simulink model "Pokus08_Display_2x2"  (Simulink 8.1)
settings: Solver=FixedStepDiscrete  StartTime=0.0  StopTime=10.0  RelTol=1e-3
libraries: simulink_extras x1, Displays_Lib x1, Computer_Library x1
settings Model: Creator=uzivatel  LastModifiedBy=uzivatel
settings DataIOCC: SignalLoggingSaveFormat=Dataset
settings OptimizationCC: ExpressionDepthLimit=128
settings DebuggingCC: FcnCallInpInsideContextMsg=EnableAllAsError
settings GRTTargetCC: CombineOutputUpdateFcns=on  GRTInterface=off

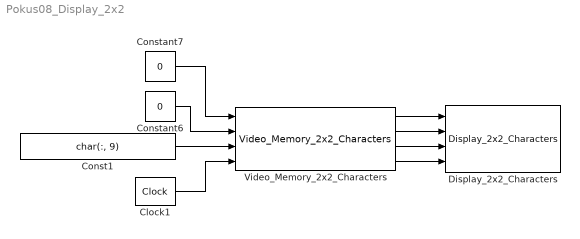
== system Pokus08_Display_2x2 ==
  Clock1 : simulink_extras/Flip Flops/Clock  period=1
  Const1 : Constant  Value=char(:, 9)  OutDataTypeStr=uint8
  Constant6 : Constant  Value=0  OutDataTypeStr=uint8
  Constant7 : Constant  Value=0  OutDataTypeStr=uint8
  Display_2x2_Characters : Displays_Lib/Displays_Lib/Display_2x2_Characters
  Video_Memory_2x2_Characters : Computer_Library/Video_Memory_2x2_Characters
  wires:
  Video_Memory_2x2_Characters/1 -> Display_2x2_Characters/1
  Video_Memory_2x2_Characters/2 -> Display_2x2_Characters/2
  Video_Memory_2x2_Characters/3 -> Display_2x2_Characters/3
  Video_Memory_2x2_Characters/4 -> Display_2x2_Characters/4
  Constant7/1 -> Video_Memory_2x2_Characters/1
  Constant6/1 -> Video_Memory_2x2_Characters/2
  Const1/1 -> Video_Memory_2x2_Characters/3
  Clock1/1 -> Video_Memory_2x2_Characters/4
